simulink subsystem "APRegler"  (R2020a)
settings: Solver=VariableStepAuto  StartTime=0.0  StopTime=10.0  RelTol=1e-3
model mask{AP=simparams.Ruhelagen(1), RegData=simparams.RegData(1)}
  mask prompts: AP "Arbeitspunkt"; RegData "APRegData"
undefined symbols (not defined in the file or in its folder): u_AP, x_AP, y_AP
settings Model: Creator=Tobias  LastModifiedBy=Tobias

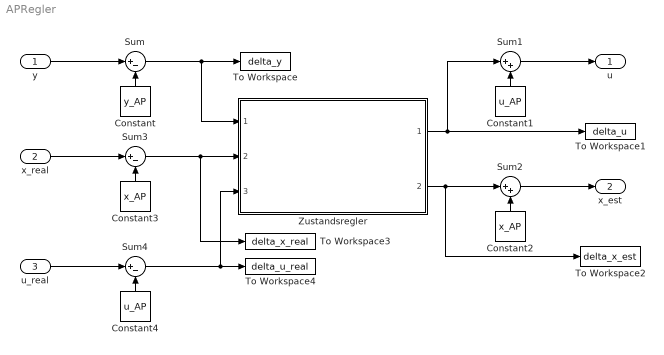
== system APRegler ==
  y : Inport
  x_real : Inport  Port=2
  u_real : Inport  Port=3
  Constant : Constant  Value=y_AP
  Constant1 : Constant  Value=u_AP
  Constant2 : Constant  Value=x_AP
  Constant3 : Constant  Value=x_AP
  Constant4 : Constant  Value=u_AP
  Sum : Sum  Inputs=|+-
  Sum1 : Sum  Inputs=|++
  Sum2 : Sum  Inputs=|++
  Sum3 : Sum  Inputs=|+-
  Sum4 : Sum  Inputs=|+-
  To Workspace : ToWorkspace  VariableName=delta_y  SaveFormat=Timeseries  SampleTime=-1
  To Workspace1 : ToWorkspace  VariableName=delta_u  SaveFormat=Timeseries  SampleTime=-1
  To Workspace2 : ToWorkspace  VariableName=delta_x_est  SaveFormat=Timeseries  SampleTime=-1
  To Workspace3 : ToWorkspace  VariableName=delta_x_real  SaveFormat=Timeseries  SampleTime=-1
  To Workspace4 : ToWorkspace  VariableName=delta_u_real  SaveFormat=Timeseries  SampleTime=-1
  Zustandsregler : Subsystem  ReferencedSubsystem=Zustandsregler  K=RegData.K  xtype=Zustandsmessung  beob=BeobData
  u : Outport
  x_est : Outport  Port=2
  wires:
  Constant4/1 -> Sum4/2
  u_real/1 -> Sum4/1
  Sum4/1 -> To Workspace4/1, Zustandsregler/3
  Zustandsregler/2 -> Sum2/1, To Workspace2/1
  Zustandsregler/1 -> To Workspace1/1, Sum1/1
  y/1 -> Sum/1
  Sum/1 -> To Workspace/1, Zustandsregler/1
  Constant/1 -> Sum/2
  Constant1/1 -> Sum1/2
  Sum1/1 -> u/1
  Sum2/1 -> x_est/1
  Constant2/1 -> Sum2/2
  Sum3/1 -> To Workspace3/1, Zustandsregler/2
  x_real/1 -> Sum3/1
  Constant3/1 -> Sum3/2
